simulink model "library_user01"  (Simulink 6.3)
settings: Solver=ode45  StartTime=0.0  StopTime=10.0  RelTol=1e-3
libraries: library01 x2
settings Model: LastModifiedBy=deissenb

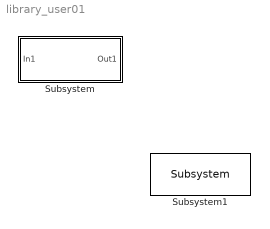
== system library_user01 ==
  Subsystem : Subsystem
  Subsystem1 : library01/Test2/Subsystem

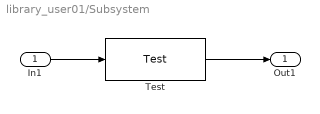
== system library_user01/Subsystem ==
  In1 : Inport
  Test : library01/Test
  Out1 : Outport
  wires:
  In1/1 -> Test/1
  Test/1 -> Out1/1
